simulink model "NetworkModelWithControl"  (R2018b)
settings: Solver=FixedStepAuto  StartTime=tStart  StopTime=tFinal  FixedStep=0.001  RelTol=1e-3
undefined symbols (not defined in the file or in its folder): bx, by, m, VelocityStarX1, VelocityStarX2, VelocityStarX3, VelocityStarX4, VelocityStarX5, VelocityStarX6, VelocityStarX7, VelocityStarX8, VelocityStarY1, VelocityStarY2, VelocityStarY3, VelocityStarY4, VelocityStarY5, VelocityStarY6, VelocityStarY7, VelocityStarY8, vx10, vx20, vx30, vx40, vx50, vx60, vx70, vx80, vy10, vy20, vy30, vy40, vy50, vy60, vy70, vy80, x10, x20, x30, x40, x50, x60, x70, x80, y10, y20, y30, y40, y50, y60, y70, y80
libraries: simulink x16
settings Model: Creator=CowUser  LastModifiedBy=CowUser

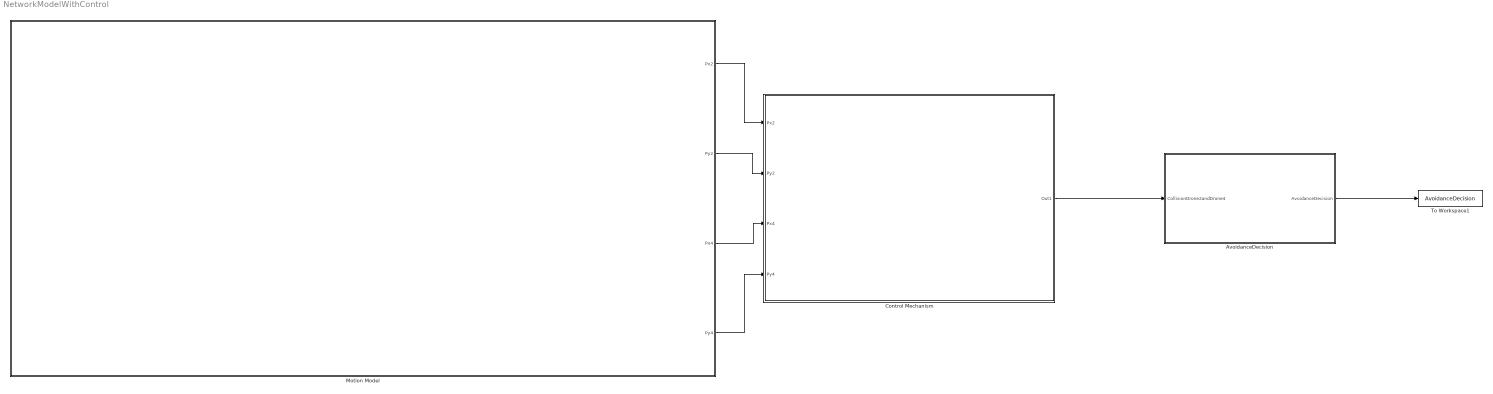
== system NetworkModelWithControl ==
  AvoidanceDecision : MATLAB Function  TreatAsAtomicUnit=on
  Control Mechanism : Subsystem
  Motion Model : Subsystem
  To Workspace1 : ToWorkspace  VariableName=AvoidanceDecision  SaveFormat=Timeseries  SampleTime=-1
  wires:
  Motion Model/1(Px2) -> Control Mechanism/1(Px2)
  Control Mechanism/1(Out1) -> AvoidanceDecision/1(CollisionDrone2andDrone4)
  AvoidanceDecision/1(AvoidanceDecision) -> To Workspace1/1
  Motion Model/2(Py2) -> Control Mechanism/2(Py2)
  Motion Model/3(Px4) -> Control Mechanism/3(Px4)
  Motion Model/4(Py4) -> Control Mechanism/4(Py4)

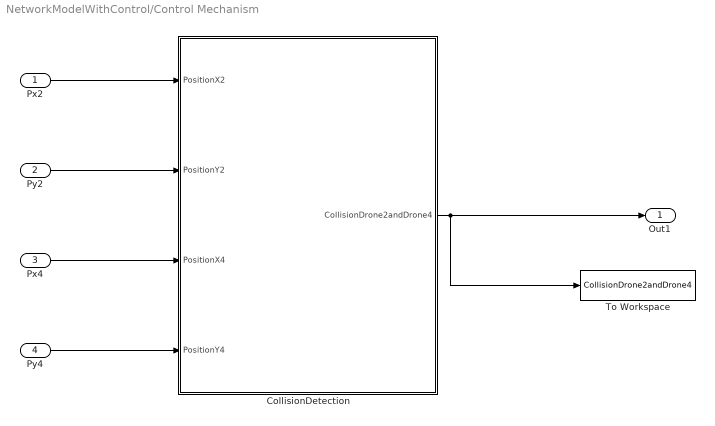
== system NetworkModelWithControl/Control Mechanism ==
  Px2 : Inport
  Py2 : Inport  Port=2
  Px4 : Inport  Port=3
  Py4 : Inport  Port=4
  CollisionDetection : MATLAB Function  TreatAsAtomicUnit=on
  To Workspace : ToWorkspace  VariableName=CollisionDrone2andDrone4  SaveFormat=Timeseries  SampleTime=-1
  Out1 : Outport
  wires:
  Px2/1 -> CollisionDetection/1(PositionX2)
  Py2/1 -> CollisionDetection/2(PositionY2)
  Px4/1 -> CollisionDetection/3(PositionX4)
  Py4/1 -> CollisionDetection/4(PositionY4)
  CollisionDetection/1(CollisionDrone2andDrone4) -> Out1/1, To Workspace/1

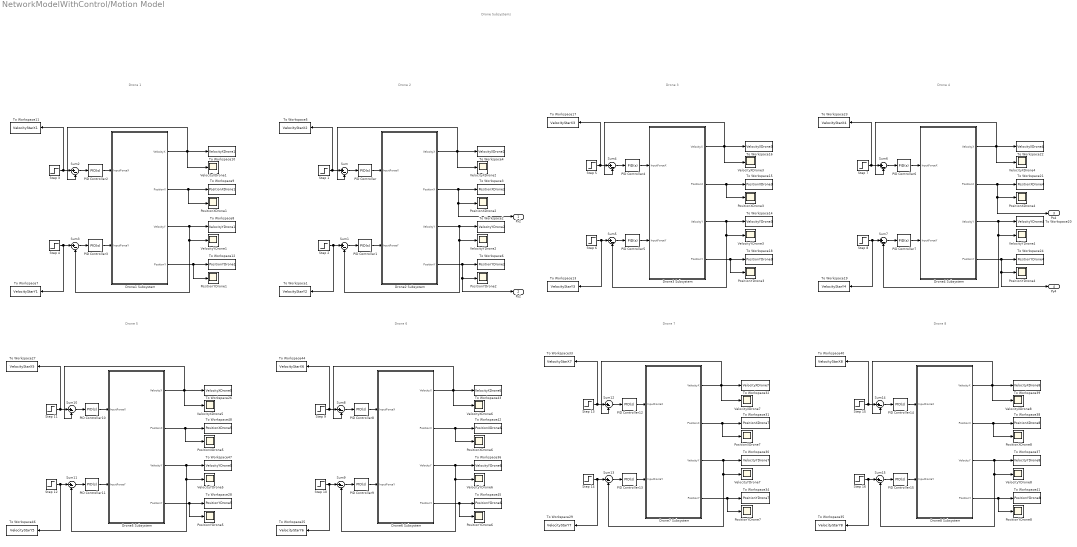
== system NetworkModelWithControl/Motion Model ==
  note: Drone 1
  note: Drone 2
  note: Drone 6
  note: Drone 3
  note: Drone Subsystems
  note: Drone 4
  note: Drone 5
  note: Drone 8
  note: Drone 7
  "Drone1 Subsystem " : Subsystem
  "Drone2 Subsystem " : Subsystem
  "Drone3 Subsystem " : Subsystem
  "Drone4 Subsystem " : Subsystem
  Drone5 Subsystem : Subsystem
  Drone6 Subsystem : Subsystem
  Drone7 Subsystem : Subsystem
  Drone8 Subsystem : Subsystem
  PID Controller{,1..15} (16 alike) : simulink/Continuous/PID Controller  Controller=PID  Form=Parallel  TimeDomain=Continuous-time  SampleTime=-1  IntegratorMethod=Forward Euler  FilterMethod=Forward Euler  ControllerParametersSource=internal  P=800  I=40  D=1  UseFilter=on  N=100  TunerSelectOption=Transfer Function Based (PID Tuner App)  InitialConditionSource=internal  InitialConditionForIntegrator=0  InitialConditionForFilter=0  DifferentiatorICPrevScaledInput=0  ExternalReset=none  TrackingMode=off  Kt=1  LimitOutput=off  UpperSaturationLimit=inf  LowerSaturationLimit=-inf  LinearizeAsGain=on  AntiWindupMode=none  Kb=1  POutMin=[]  POutMax=[]  IOutMin=[]  IOutMax=[]  DOutMin=[]  DOutMax=[]  NOutMin=[]  NOutMax=[]  SumOutMin=[]  SumOutMax=[]  SaturationOutMin=[]  SaturationOutMax=[]  PParamMin=[]  PParamMax=[]  IParamMin=[]  IParamMax=[]  DParamMin=[]  DParamMax=[]  NParamMin=[]  NParamMax=[]  KbParamMin=[]  KbParamMax=[]  KtParamMin=[]  KtParamMax=[]  KbOutMin=[]  KbOutMax=[]  KtOutMin=[]  KtOutMax=[]  IntegratorOutMin=[]  IntegratorOutMax=[]  FilterOutMin=[]  FilterOutMax=[]  SumI1OutMin=[]  SumI1OutMax=[]  SumI2OutMin=[]  SumI2OutMax=[]  SumI3OutMin=[]  SumI3OutMax=[]  SumI4OutMin=[]  SumI4OutMax=[]  SumDOutMin=[]  SumDOutMax=[]  DifferentiatorOutMin=[]  DifferentiatorOutMax=[]  FilterDiffOutCoefMin=[]  FilterDiffOutCoefMax=[]  ReciprocalOutMin=[]  ReciprocalOutMax=[]  SumDenOutMin=[]  SumDenOutMax=[]  SumNumOutMin=[]  SumNumOutMax=[]  DivideOutMin=[]  DivideOutMax=[]  IntegratorContinuousStateAttributes=''  IntegratorStateMustResolveToSignalObject=off  IntegratorRTWStateStorageClass=Auto  FilterContinuousStateAttributes=''  FilterStateMustResolveToSignalObject=off  FilterRTWStateStorageClass=Auto  ParallelPVariant=InternalParameters  IdealPVariant=Disabled  IVariant=InternalParameters  DVariant=InternalParameters  IntegratorVariant=Continuous  SatVariant=Disabled  AWVariant=Passthrough  PCopyVariant=Disabled  TRVariant=Disabled  FdbkBlocksVariant=Forward  IdealPFdbkVariant=Disabled  SatFdbkVariant=Disabled  DerivativeFilterVariant=ContFilter  NVariant=InternalParameters  NCopyVariant=Disabled  FilterICVariant=InternalICsFilter  IntegratorICVariant=InternalICs  ExternalResetVariant=Disabled  TRSumVariant=Passthrough  SumFdbkVariant=Disabled  SumVariant=Sum_PID
  PositionXDrone{1..8} (8 alike) : Scope
  PositionYDrone{1..8} (8 alike) : Scope
  Step 1 : Step  Time=0  After=VelocityStarX2  SampleTime=0
  Step 10 : Step  Time=0  After=VelocityStarY6  SampleTime=0
  Step 11 : Step  Time=0  After=VelocityStarX5  SampleTime=0
  Step 12 : Step  Time=0  After=VelocityStarY5  SampleTime=0
  Step 13 : Step  Time=0  After=VelocityStarX7  SampleTime=0
  Step 14 : Step  Time=0  After=VelocityStarY7  SampleTime=0
  Step 15 : Step  Time=0  After=VelocityStarX8  SampleTime=0
  Step 16 : Step  Time=0  After=VelocityStarY8  SampleTime=0
  Step 2 : Step  Time=0  After=VelocityStarY2  SampleTime=0
  Step 3 : Step  Time=0  After=VelocityStarX1  SampleTime=0
  Step 4 : Step  Time=0  After=VelocityStarY1  SampleTime=0
  Step 5 : Step  Time=0  After=VelocityStarX3  SampleTime=0
  Step 6 : Step  Time=0  After=VelocityStarY3  SampleTime=0
  Step 7 : Step  Time=0  After=VelocityStarX4  SampleTime=0
  Step 8 : Step  Time=0  After=VelocityStarY4  SampleTime=0
  Step 9 : Step  Time=0  After=VelocityStarX6  SampleTime=0
  Sum{,1..15} (16 alike) : Sum  Inputs=|+-
  To Workspace1 : ToWorkspace  VariableName=VelocityStarY2  SampleTime=-1
  To Workspace10 : ToWorkspace  VariableName=VelocityXDrone1  SampleTime=-1
  To Workspace11 : ToWorkspace  VariableName=VelocityStarX1  SampleTime=-1
  To Workspace12 : ToWorkspace  VariableName=PositionYDrone1  SampleTime=-1
  To Workspace13 : ToWorkspace  VariableName=VelocityStarY3  SampleTime=-1
  To Workspace14 : ToWorkspace  VariableName=VelocityYDrone3  SampleTime=-1
  To Workspace15 : ToWorkspace  VariableName=PositionXDrone3  SampleTime=-1
  To Workspace16 : ToWorkspace  VariableName=VelocityXDrone3  SampleTime=-1
  To Workspace17 : ToWorkspace  VariableName=VelocityStarX3  SampleTime=-1
  To Workspace18 : ToWorkspace  VariableName=PositionYDrone3  SampleTime=-1
  To Workspace19 : ToWorkspace  VariableName=VelocityStarY4  SampleTime=-1
  To Workspace2 : ToWorkspace  VariableName=VelocityYDrone2  SampleTime=-1
  To Workspace20 : ToWorkspace  VariableName=VelocityYDrone4  SampleTime=-1
  To Workspace21 : ToWorkspace  VariableName=PositionXDrone4  SampleTime=-1
  To Workspace22 : ToWorkspace  VariableName=VelocityXDrone4  SampleTime=-1
  To Workspace23 : ToWorkspace  VariableName=VelocityStarX4  SampleTime=-1
  To Workspace24 : ToWorkspace  VariableName=PositionYDrone4  SampleTime=-1
  To Workspace25 : ToWorkspace  VariableName=VelocityStarY6  SampleTime=-1
  To Workspace26 : ToWorkspace  VariableName=VelocityXDrone5  SampleTime=-1
  To Workspace27 : ToWorkspace  VariableName=VelocityStarX5  SampleTime=-1
  To Workspace28 : ToWorkspace  VariableName=PositionYDrone5  SampleTime=-1
  To Workspace29 : ToWorkspace  VariableName=VelocityStarY7  SampleTime=-1
  To Workspace3 : ToWorkspace  VariableName=PositionXDrone2  SampleTime=-1
  To Workspace30 : ToWorkspace  VariableName=VelocityYDrone7  SampleTime=-1
  To Workspace31 : ToWorkspace  VariableName=PositionXDrone7  SampleTime=-1
  To Workspace32 : ToWorkspace  VariableName=VelocityXDrone7  SampleTime=-1
  To Workspace33 : ToWorkspace  VariableName=VelocityStarX7  SampleTime=-1
  To Workspace34 : ToWorkspace  VariableName=PositionYDrone7  SampleTime=-1
  To Workspace35 : ToWorkspace  VariableName=VelocityStarY8  SampleTime=-1
  To Workspace36 : ToWorkspace  VariableName=VelocityYDrone6  SampleTime=-1
  To Workspace37 : ToWorkspace  VariableName=VelocityYDrone8  SampleTime=-1
  To Workspace38 : ToWorkspace  VariableName=PositionXDrone8  SampleTime=-1
  To Workspace39 : ToWorkspace  VariableName=VelocityXDrone8  SampleTime=-1
  To Workspace4 : ToWorkspace  VariableName=VelocityXDrone2  SampleTime=-1
  To Workspace40 : ToWorkspace  VariableName=VelocityStarX8  SampleTime=-1
  To Workspace41 : ToWorkspace  VariableName=PositionYDrone8  SampleTime=-1
  To Workspace42 : ToWorkspace  VariableName=PositionXDrone6  SampleTime=-1
  To Workspace43 : ToWorkspace  VariableName=VelocityXDrone6  SampleTime=-1
  To Workspace44 : ToWorkspace  VariableName=VelocityStarX6  SampleTime=-1
  To Workspace45 : ToWorkspace  VariableName=PositionYDrone6  SampleTime=-1
  To Workspace46 : ToWorkspace  VariableName=VelocityStarY5  SampleTime=-1
  To Workspace47 : ToWorkspace  VariableName=VelocityYDrone5  SampleTime=-1
  To Workspace48 : ToWorkspace  VariableName=PositionXDrone5  SampleTime=-1
  To Workspace5 : ToWorkspace  VariableName=VelocityStarX2  SampleTime=-1
  To Workspace6 : ToWorkspace  VariableName=PositionYDrone2  SampleTime=-1
  To Workspace7 : ToWorkspace  VariableName=VelocityStarY1  SampleTime=-1
  To Workspace8 : ToWorkspace  VariableName=VelocityYDrone1  SampleTime=-1
  To Workspace9 : ToWorkspace  VariableName=PositionXDrone1  SampleTime=-1
  VelocityXDrone{1..8} (8 alike) : Scope
  VelocityYDrone{1..8} (8 alike) : Scope
  Px2 : Outport
  Py2 : Outport  Port=2
  Px4 : Outport  Port=3
  Py4 : Outport  Port=4
  wires:
  Sum/1 -> PID Controller/1
  "Drone2 Subsystem "/3(VelocityY) -> Sum1/2, VelocityYDrone2/1, To Workspace2/1
  Sum1/1 -> PID Controller1/1
  PID Controller/1 -> "Drone2 Subsystem "/1(InputForceX)
  "Drone1 Subsystem "/4(PositionY) -> PositionYDrone1/1, To Workspace12/1
  "Drone2 Subsystem "/4(PositionY) -> Py2/1, PositionYDrone2/1, To Workspace6/1
  PID Controller7/1 -> "Drone4 Subsystem "/2(InputForceY)
  Step 16/1 -> To Workspace35/1, Sum15/1
  Step 14/1 -> To Workspace29/1, Sum13/1
  Step 12/1 -> To Workspace46/1, Sum11/1
  "Drone2 Subsystem "/2(PositionX) -> Px2/1, PositionXDrone2/1, To Workspace3/1
  Sum11/1 -> PID Controller11/1
  PID Controller6/1 -> "Drone4 Subsystem "/1(InputForceX)
  Drone6 Subsystem/1(VelocityX) -> Sum8/2, To Workspace43/1, VelocityXDrone6/1
  Sum15/1 -> PID Controller15/1
  PID Controller8/1 -> Drone6 Subsystem/1(InputForceX)
  Step 2/1 -> To Workspace1/1, Sum1/1
  Step 9/1 -> Sum8/1, To Workspace44/1
  Step 13/1 -> Sum12/1, To Workspace33/1
  PID Controller14/1 -> Drone8 Subsystem/1(InputForceX)
  Drone6 Subsystem/3(VelocityY) -> Sum9/2, VelocityYDrone6/1, To Workspace36/1
  "Drone3 Subsystem "/2(PositionX) -> PositionXDrone3/1, To Workspace15/1
  Sum6/1 -> PID Controller6/1
  Drone6 Subsystem/2(PositionX) -> PositionXDrone6/1, To Workspace42/1
  Drone8 Subsystem/2(PositionX) -> PositionXDrone8/1, To Workspace38/1
  Drone7 Subsystem/3(VelocityY) -> Sum13/2, VelocityYDrone7/1, To Workspace30/1
  Drone8 Subsystem/3(VelocityY) -> Sum15/2, VelocityYDrone8/1, To Workspace37/1
  Sum4/1 -> PID Controller4/1
  Drone7 Subsystem/2(PositionX) -> PositionXDrone7/1, To Workspace31/1
  PID Controller12/1 -> Drone7 Subsystem/1(InputForceX)
  PID Controller1/1 -> "Drone2 Subsystem "/2(InputForceY)
  "Drone2 Subsystem "/1(VelocityX) -> Sum/2, To Workspace4/1, VelocityXDrone2/1
  Drone5 Subsystem/2(PositionX) -> PositionXDrone5/1, To Workspace48/1
  Sum13/1 -> PID Controller13/1
  "Drone4 Subsystem "/4(PositionY) -> Py4/1, PositionYDrone4/1, To Workspace24/1
  Drone7 Subsystem/4(PositionY) -> PositionYDrone7/1, To Workspace34/1
  "Drone4 Subsystem "/3(VelocityY) -> Sum7/2, VelocityYDrone4/1, To Workspace20/1
  Step 5/1 -> Sum4/1, To Workspace17/1
  "Drone4 Subsystem "/1(VelocityX) -> Sum6/2, To Workspace22/1, VelocityXDrone4/1
  Step 7/1 -> Sum6/1, To Workspace23/1
  Sum7/1 -> PID Controller7/1
  Step 8/1 -> To Workspace19/1, Sum7/1
  PID Controller5/1 -> "Drone3 Subsystem "/2(InputForceY)
  PID Controller15/1 -> Drone8 Subsystem/2(InputForceY)
  "Drone3 Subsystem "/4(PositionY) -> PositionYDrone3/1, To Workspace18/1
  "Drone1 Subsystem "/1(VelocityX) -> To Workspace10/1, VelocityXDrone1/1, Sum2/2
  Step 4/1 -> To Workspace7/1, Sum3/1
  PID Controller3/1 -> "Drone1 Subsystem "/2(InputForceY)
  "Drone3 Subsystem "/3(VelocityY) -> Sum5/2, VelocityYDrone3/1, To Workspace14/1
  Sum2/1 -> PID Controller2/1
  "Drone1 Subsystem "/3(VelocityY) -> Sum3/2, VelocityYDrone1/1, To Workspace8/1
  Step 1/1 -> Sum/1, To Workspace5/1
  Drone5 Subsystem/4(PositionY) -> PositionYDrone5/1, To Workspace28/1
  PID Controller10/1 -> Drone5 Subsystem/1(InputForceX)
  Sum9/1 -> PID Controller9/1
  Step 3/1 -> Sum2/1, To Workspace11/1
  Drone8 Subsystem/4(PositionY) -> PositionYDrone8/1, To Workspace41/1
  Sum10/1 -> PID Controller10/1
  PID Controller11/1 -> Drone5 Subsystem/2(InputForceY)
  Sum3/1 -> PID Controller3/1
  Step 6/1 -> To Workspace13/1, Sum5/1
  Step 11/1 -> Sum10/1, To Workspace27/1
  Sum14/1 -> PID Controller14/1
  Step 10/1 -> To Workspace25/1, Sum9/1
  PID Controller13/1 -> Drone7 Subsystem/2(InputForceY)
  "Drone1 Subsystem "/2(PositionX) -> PositionXDrone1/1, To Workspace9/1
  Drone5 Subsystem/3(VelocityY) -> Sum11/2, VelocityYDrone5/1, To Workspace47/1
  Sum5/1 -> PID Controller5/1
  Sum12/1 -> PID Controller12/1
  PID Controller4/1 -> "Drone3 Subsystem "/1(InputForceX)
  "Drone4 Subsystem "/2(PositionX) -> Px4/1, PositionXDrone4/1, To Workspace21/1
  PID Controller9/1 -> Drone6 Subsystem/2(InputForceY)
  Drone6 Subsystem/4(PositionY) -> PositionYDrone6/1, To Workspace45/1
  Drone7 Subsystem/1(VelocityX) -> Sum12/2, To Workspace32/1, VelocityXDrone7/1
  PID Controller2/1 -> "Drone1 Subsystem "/1(InputForceX)
  Step 15/1 -> Sum14/1, To Workspace40/1
  Drone8 Subsystem/1(VelocityX) -> Sum14/2, To Workspace39/1, VelocityXDrone8/1
  Drone5 Subsystem/1(VelocityX) -> To Workspace26/1, VelocityXDrone5/1, Sum10/2
  "Drone3 Subsystem "/1(VelocityX) -> Sum4/2, To Workspace16/1, VelocityXDrone3/1
  Sum8/1 -> PID Controller8/1

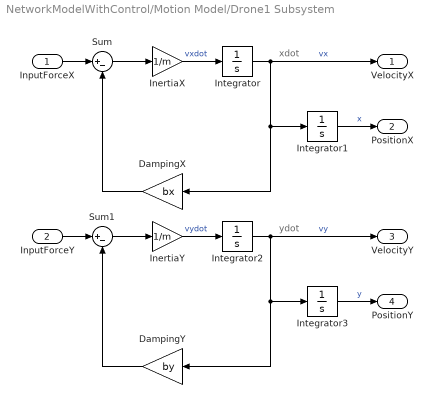
== system NetworkModelWithControl/Motion Model/Drone1 Subsystem  ==
  note: xdot
  note: ydot
  InputForceX : Inport
  InputForceY : Inport  Port=2
  "DampingX " : Gain  Gain=bx
  DampingY : Gain  Gain=by
  InertiaX : Gain  Gain=1/m
  InertiaY : Gain  Gain=1/m
  Integrator : Integrator  InitialCondition=vx10
  Integrator1 : Integrator  InitialCondition=x10
  Integrator2 : Integrator  InitialCondition=vy10
  Integrator3 : Integrator  InitialCondition=y10
  Sum : Sum  Inputs=|+-
  Sum1 : Sum  Inputs=|+-
  VelocityX : Outport
  PositionX : Outport  Port=2
  VelocityY : Outport  Port=3
  PositionY : Outport  Port=4
  wires:
  InputForceX/1 -> Sum/1
  InertiaX/1 -> Integrator/1  "vxdot"
  Sum/1 -> InertiaX/1
  Integrator/1 -> VelocityX/1, Integrator1/1, "DampingX "/1  "vx"
  "DampingX "/1 -> Sum/2
  Integrator1/1 -> PositionX/1  "x"
  DampingY/1 -> Sum1/2
  Sum1/1 -> InertiaY/1
  InertiaY/1 -> Integrator2/1  "vydot"
  Integrator3/1 -> PositionY/1  "y"
  InputForceY/1 -> Sum1/1
  Integrator2/1 -> VelocityY/1, Integrator3/1, DampingY/1  "vy"

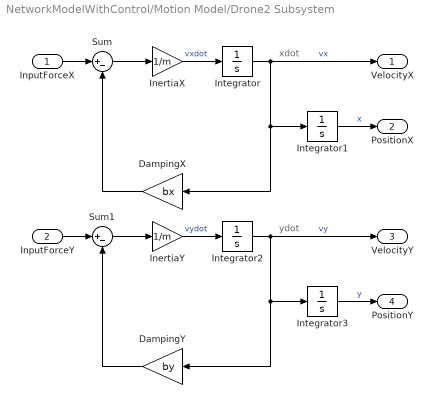
== system NetworkModelWithControl/Motion Model/Drone2 Subsystem  ==
  note: xdot
  note: ydot
  InputForceX : Inport
  InputForceY : Inport  Port=2
  "DampingX " : Gain  Gain=bx
  DampingY : Gain  Gain=by
  InertiaX : Gain  Gain=1/m
  InertiaY : Gain  Gain=1/m
  Integrator : Integrator  InitialCondition=vx20
  Integrator1 : Integrator  InitialCondition=x20
  Integrator2 : Integrator  InitialCondition=vy20
  Integrator3 : Integrator  InitialCondition=y20
  Sum : Sum  Inputs=|+-
  Sum1 : Sum  Inputs=|+-
  VelocityX : Outport
  PositionX : Outport  Port=2
  VelocityY : Outport  Port=3
  PositionY : Outport  Port=4
  wires:
  InputForceX/1 -> Sum/1
  InertiaX/1 -> Integrator/1  "vxdot"
  Sum/1 -> InertiaX/1
  Integrator/1 -> VelocityX/1, Integrator1/1, "DampingX "/1  "vx"
  "DampingX "/1 -> Sum/2
  Integrator1/1 -> PositionX/1  "x"
  DampingY/1 -> Sum1/2
  Sum1/1 -> InertiaY/1
  InertiaY/1 -> Integrator2/1  "vydot"
  Integrator3/1 -> PositionY/1  "y"
  InputForceY/1 -> Sum1/1
  Integrator2/1 -> VelocityY/1, Integrator3/1, DampingY/1  "vy"

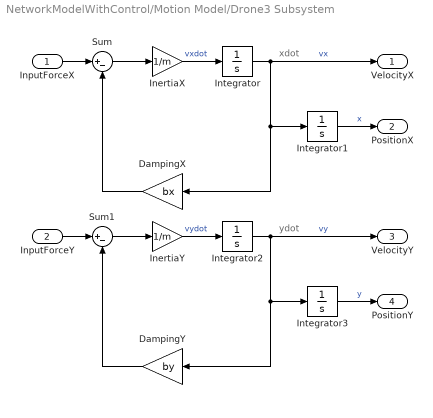
== system NetworkModelWithControl/Motion Model/Drone3 Subsystem  ==
  note: xdot
  note: ydot
  InputForceX : Inport
  InputForceY : Inport  Port=2
  "DampingX " : Gain  Gain=bx
  DampingY : Gain  Gain=by
  InertiaX : Gain  Gain=1/m
  InertiaY : Gain  Gain=1/m
  Integrator : Integrator  InitialCondition=vx30
  Integrator1 : Integrator  InitialCondition=x30
  Integrator2 : Integrator  InitialCondition=vy30
  Integrator3 : Integrator  InitialCondition=y30
  Sum : Sum  Inputs=|+-
  Sum1 : Sum  Inputs=|+-
  VelocityX : Outport
  PositionX : Outport  Port=2
  VelocityY : Outport  Port=3
  PositionY : Outport  Port=4
  wires:
  InputForceX/1 -> Sum/1
  InertiaX/1 -> Integrator/1  "vxdot"
  Sum/1 -> InertiaX/1
  Integrator/1 -> VelocityX/1, Integrator1/1, "DampingX "/1  "vx"
  "DampingX "/1 -> Sum/2
  Integrator1/1 -> PositionX/1  "x"
  DampingY/1 -> Sum1/2
  Sum1/1 -> InertiaY/1
  InertiaY/1 -> Integrator2/1  "vydot"
  Integrator3/1 -> PositionY/1  "y"
  InputForceY/1 -> Sum1/1
  Integrator2/1 -> VelocityY/1, Integrator3/1, DampingY/1  "vy"

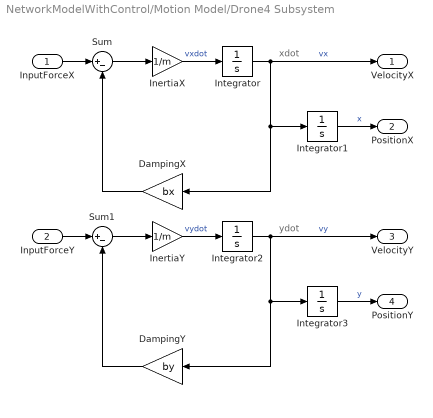
== system NetworkModelWithControl/Motion Model/Drone4 Subsystem  ==
  note: xdot
  note: ydot
  InputForceX : Inport
  InputForceY : Inport  Port=2
  "DampingX " : Gain  Gain=bx
  DampingY : Gain  Gain=by
  InertiaX : Gain  Gain=1/m
  InertiaY : Gain  Gain=1/m
  Integrator : Integrator  InitialCondition=vx40
  Integrator1 : Integrator  InitialCondition=x40
  Integrator2 : Integrator  InitialCondition=vy40
  Integrator3 : Integrator  InitialCondition=y40
  Sum : Sum  Inputs=|+-
  Sum1 : Sum  Inputs=|+-
  VelocityX : Outport
  PositionX : Outport  Port=2
  VelocityY : Outport  Port=3
  PositionY : Outport  Port=4
  wires:
  InputForceX/1 -> Sum/1
  InertiaX/1 -> Integrator/1  "vxdot"
  Sum/1 -> InertiaX/1
  Integrator/1 -> VelocityX/1, Integrator1/1, "DampingX "/1  "vx"
  "DampingX "/1 -> Sum/2
  Integrator1/1 -> PositionX/1  "x"
  DampingY/1 -> Sum1/2
  Sum1/1 -> InertiaY/1
  InertiaY/1 -> Integrator2/1  "vydot"
  Integrator3/1 -> PositionY/1  "y"
  InputForceY/1 -> Sum1/1
  Integrator2/1 -> VelocityY/1, Integrator3/1, DampingY/1  "vy"

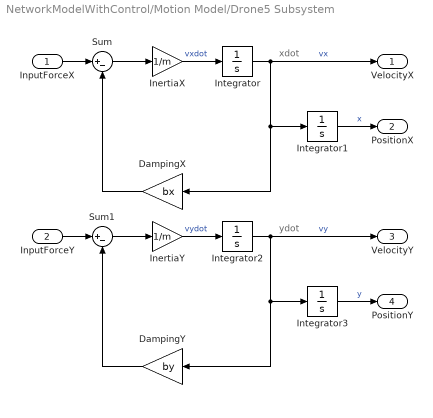
== system NetworkModelWithControl/Motion Model/Drone5 Subsystem ==
  note: xdot
  note: ydot
  InputForceX : Inport
  InputForceY : Inport  Port=2
  "DampingX " : Gain  Gain=bx
  DampingY : Gain  Gain=by
  InertiaX : Gain  Gain=1/m
  InertiaY : Gain  Gain=1/m
  Integrator : Integrator  InitialCondition=vx50
  Integrator1 : Integrator  InitialCondition=x50
  Integrator2 : Integrator  InitialCondition=vy50
  Integrator3 : Integrator  InitialCondition=y50
  Sum : Sum  Inputs=|+-
  Sum1 : Sum  Inputs=|+-
  VelocityX : Outport
  PositionX : Outport  Port=2
  VelocityY : Outport  Port=3
  PositionY : Outport  Port=4
  wires:
  InputForceX/1 -> Sum/1
  InertiaX/1 -> Integrator/1  "vxdot"
  Sum/1 -> InertiaX/1
  Integrator/1 -> VelocityX/1, Integrator1/1, "DampingX "/1  "vx"
  "DampingX "/1 -> Sum/2
  Integrator1/1 -> PositionX/1  "x"
  DampingY/1 -> Sum1/2
  Sum1/1 -> InertiaY/1
  InertiaY/1 -> Integrator2/1  "vydot"
  Integrator3/1 -> PositionY/1  "y"
  InputForceY/1 -> Sum1/1
  Integrator2/1 -> VelocityY/1, Integrator3/1, DampingY/1  "vy"

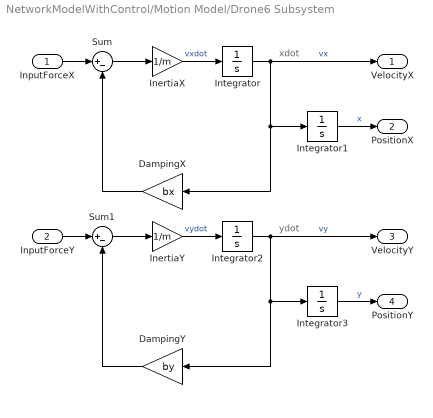
== system NetworkModelWithControl/Motion Model/Drone6 Subsystem ==
  note: xdot
  note: ydot
  InputForceX : Inport
  InputForceY : Inport  Port=2
  "DampingX " : Gain  Gain=bx
  DampingY : Gain  Gain=by
  InertiaX : Gain  Gain=1/m
  InertiaY : Gain  Gain=1/m
  Integrator : Integrator  InitialCondition=vx60
  Integrator1 : Integrator  InitialCondition=x60
  Integrator2 : Integrator  InitialCondition=vy60
  Integrator3 : Integrator  InitialCondition=y60
  Sum : Sum  Inputs=|+-
  Sum1 : Sum  Inputs=|+-
  VelocityX : Outport
  PositionX : Outport  Port=2
  VelocityY : Outport  Port=3
  PositionY : Outport  Port=4
  wires:
  InputForceX/1 -> Sum/1
  InertiaX/1 -> Integrator/1  "vxdot"
  Sum/1 -> InertiaX/1
  Integrator/1 -> VelocityX/1, Integrator1/1, "DampingX "/1  "vx"
  "DampingX "/1 -> Sum/2
  Integrator1/1 -> PositionX/1  "x"
  DampingY/1 -> Sum1/2
  Sum1/1 -> InertiaY/1
  InertiaY/1 -> Integrator2/1  "vydot"
  Integrator3/1 -> PositionY/1  "y"
  InputForceY/1 -> Sum1/1
  Integrator2/1 -> VelocityY/1, Integrator3/1, DampingY/1  "vy"

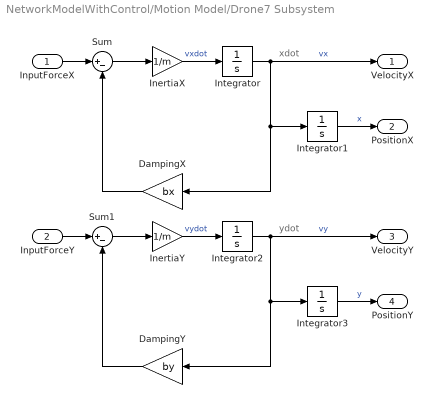
== system NetworkModelWithControl/Motion Model/Drone7 Subsystem ==
  note: xdot
  note: ydot
  InputForceX : Inport
  InputForceY : Inport  Port=2
  "DampingX " : Gain  Gain=bx
  DampingY : Gain  Gain=by
  InertiaX : Gain  Gain=1/m
  InertiaY : Gain  Gain=1/m
  Integrator : Integrator  InitialCondition=vx70
  Integrator1 : Integrator  InitialCondition=x70
  Integrator2 : Integrator  InitialCondition=vy70
  Integrator3 : Integrator  InitialCondition=y70
  Sum : Sum  Inputs=|+-
  Sum1 : Sum  Inputs=|+-
  VelocityX : Outport
  PositionX : Outport  Port=2
  VelocityY : Outport  Port=3
  PositionY : Outport  Port=4
  wires:
  InputForceX/1 -> Sum/1
  InertiaX/1 -> Integrator/1  "vxdot"
  Sum/1 -> InertiaX/1
  Integrator/1 -> VelocityX/1, Integrator1/1, "DampingX "/1  "vx"
  "DampingX "/1 -> Sum/2
  Integrator1/1 -> PositionX/1  "x"
  DampingY/1 -> Sum1/2
  Sum1/1 -> InertiaY/1
  InertiaY/1 -> Integrator2/1  "vydot"
  Integrator3/1 -> PositionY/1  "y"
  InputForceY/1 -> Sum1/1
  Integrator2/1 -> VelocityY/1, Integrator3/1, DampingY/1  "vy"

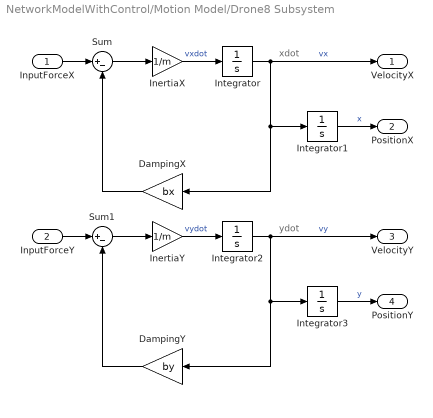
== system NetworkModelWithControl/Motion Model/Drone8 Subsystem ==
  note: xdot
  note: ydot
  InputForceX : Inport
  InputForceY : Inport  Port=2
  "DampingX " : Gain  Gain=bx
  DampingY : Gain  Gain=by
  InertiaX : Gain  Gain=1/m
  InertiaY : Gain  Gain=1/m
  Integrator : Integrator  InitialCondition=vx80
  Integrator1 : Integrator  InitialCondition=x80
  Integrator2 : Integrator  InitialCondition=vy80
  Integrator3 : Integrator  InitialCondition=y80
  Sum : Sum  Inputs=|+-
  Sum1 : Sum  Inputs=|+-
  VelocityX : Outport
  PositionX : Outport  Port=2
  VelocityY : Outport  Port=3
  PositionY : Outport  Port=4
  wires:
  InputForceX/1 -> Sum/1
  InertiaX/1 -> Integrator/1  "vxdot"
  Sum/1 -> InertiaX/1
  Integrator/1 -> VelocityX/1, Integrator1/1, "DampingX "/1  "vx"
  "DampingX "/1 -> Sum/2
  Integrator1/1 -> PositionX/1  "x"
  DampingY/1 -> Sum1/2
  Sum1/1 -> InertiaY/1
  InertiaY/1 -> Integrator2/1  "vydot"
  Integrator3/1 -> PositionY/1  "y"
  InputForceY/1 -> Sum1/1
  Integrator2/1 -> VelocityY/1, Integrator3/1, DampingY/1  "vy"

== matlab function NetworkModelWithControl/AvoidanceDecision ==
  data: AvoidanceDecision output; CollisionDrone2andDrone4 input
function AvoidanceDecision = AvoidanceDecision(CollisionDrone2andDrone4)



%% Conflict Detection
  
        if (CollisionDrone2andDrone4 == 1)% If there is a collsiion
        
            
                % 1)	Right-of-way Rule (to tackle M-1)
                
                        AvoidanceDecision = 1;
                
                % 2)	Priority Rule (to tackle M-2)
                
%                        AvoidanceDecision = 2; 
                
                % 3)	High Speed Rule (to tackle M-3)
                        
%                        AvoidanceDecision = 3; 
        else 
            
            AvoidanceDecision = 0 ; % No need to make an Avoidance Decision
         
        end
          
end

== matlab function NetworkModelWithControl/Control Mechanism/CollisionDetection ==
  data: PositionX2 input; PositionY2 input; PositionX4 input; PositionY4 input; CollisionDrone2andDrone4 output
function CollisionDrone2andDrone4 = CollisionDetection(PositionX2, PositionY2, PositionX4, PositionY4)

%% Conflict Detection
coder.extrinsic('warning') 

% No more than one agent is allowed in the crtical zone
    r = 1; % Radius of the critical zone
    
        if (sqrt(PositionX2^2 + PositionY2^2)<= r)&& (sqrt(PositionX4^2 + PositionY4^2)<= r)% Compare the position coordinates of the drones at a given time k
        
            CollisionDrone2andDrone4 = 1
                
        end
          
end
